simulink model "control_nonlinear"  (R2025a)
settings: Solver=VariableStepAuto  StartTime=0.0  StopTime=10.0  RelTol=1e-3
values from neighbouring files (symbols this model uses):
  dth1_0 = casos(k, 4)    [main.m]
  dth2_0 = casos(k, 6)    [main.m]
  dxc_0 = casos(k, 2)    [main.m]
  g = 9.8    [main.m]
  l1 = 0.42    [main.m]
  l2 = 0.191    [main.m]
  m1 = 3.0    (= 3)    [main.m]
  m2 = 3.3    [main.m]
  Mc = 5.5    [main.m]
  th1_0 = casos(k, 3)    [main.m]
  th2_0 = casos(k, 5)    [main.m]
  xc_0 = casos(k, 1)    [main.m]
undefined symbols (not defined in the file or in its folder): K, K_cancel, T, X, Y, Z
libraries: sm_lib x43, nesl_utility x10
(part 1 of 2)
settings Model: Creator=amoralesma  LastModifiedBy=amoralesma

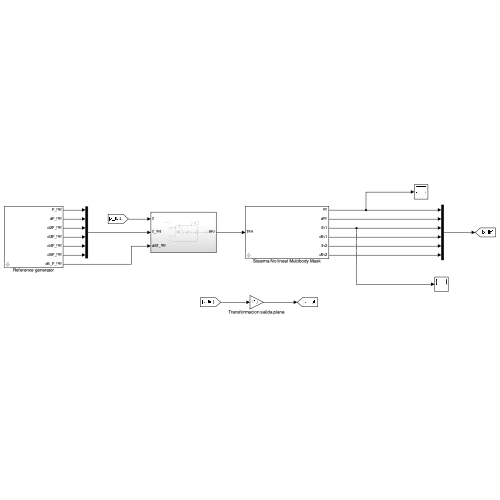
[thumbnail: Simulink's stored preview of the top-level diagram]
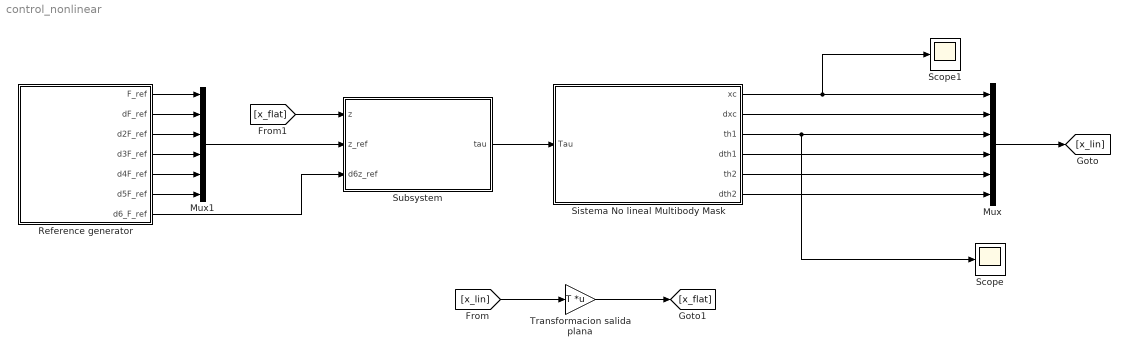
== system control_nonlinear ==
  Mux : Mux  Inputs=6
  Mux1 : Mux  Inputs=6
  Reference generator : Subsystem  mask(Generador señales de referencia carro y dos pendulos.){z2f=T, xc_in=xc_0, dxc_in=dxc_0, th1_in=th1_0, dth1_in=dth1_0, th2_in=th2_0, dth2_in=dth2_0, tf_=8, xc_f=-3, ref_config_sel=Suave quinta derivada (polinomio orden 11)}
      mask prompts: z2f "Matriz (6x6) transformación estados a salida plana"; tf_ "Tiempo final [s]"; xc_f "Posición final carro [m]"; ref_config_sel "Suavidad referencia"
      mask help: Este bloque realiza el planeamiento de las señales de referencia de las salida plana y sus derivadas, para un sistema de sexto orden, que corresponde a un carro con dos pendulos. Utiliza teoría de planitud diferencial y información de las condiciones iniciales y finales del sistema.
      mask init:
      | MaskNames = get_param(gcb,'MaskNames');
      | MaskVal = get_param(gcb,'MaskValues');
      | MaskObj = get_param(gcb,'MaskObject');
      | Model_folder=fileparts(which(gcs));
      | 
      | for ii_msk=1:length(MaskObj.Parameters)
      |     Obj_ii=MaskObj.Parameters(ii_msk);
      |     switch Obj_ii.Type
      |         case 'popup'
      |             eval([Obj_ii.Name,'=''',Obj_ii.Value,''';']);
      |             idx=find(strcmp(Obj_ii.TypeOptions, Obj_ii.Value));
      |             eval([Obj_ii.Name,'_idx=',num2str(idx),';']);
      |             clear idx  
      |         case 'edit'
      |             try
      |                 eval([MaskNames{ii_msk},'=',MaskVal{ii_msk},';']);
      |             catch
      |                 Work_space_vars=MaskObj.getWorkspaceVariables;
      |                idx_value=find(strcmp(MaskNames{ii_msk},{Work_space_vars.Name}));
      |                eval([MaskNames{ii_msk},'=Work_space_vars(idx_value).Value;'])
      |             end
      | 
      |         case 'checkbox'
      | 
      |             if strcmp(MaskVal{ii_msk},'on')
      |                 eval([MaskNames{ii_msk},'=true;']);
      |             else
      |                 eval([MaskNames{ii_msk},'=false;']);
      |             end
      | 
      |         case 'customtable'
      | 
      |             eval([MaskNames{ii_msk},'=',Obj_ii.Value,';']);
      |             eval([MaskNames{ii_msk},'_par=Obj_ii;']);
      |             eval([MaskNames{ii_msk},'_ctr=Obj_ii.DialogControl;']);
      | 
      |         case 'listbox'
      | 
      |             Options=Obj_ii.TypeOptions;
      |             if ~isempty(Obj_ii.TypeOptions)
      |                 if ~strcmp(Obj_ii.Value,'<empty>')
      |                     eval(['Val=',Obj_ii.Value,';'])
      |                     eval([MaskNames{ii_msk},'_idx=ismember(Options,Val);']);
      |                     eval([MaskNames{ii_msk},'=Options(ismember(Options,Val));']);
      |                 else
      |                     Val='<empty>';
      |                     eval([MaskNames{ii_msk},'_idx=ismember(Options,Val);']);
      |                     eval([MaskNames{ii_msk},'=Options(ismember(Options,Val));']);
      | 
      |                 end
      |             end
      | 
      |         case 'spinbox'
      | 
      |           
      |             eval([MaskNames{ii_msk},'=',MaskVal{ii_msk},';']);
      | 
      |     end      
      | end
      | 
      | 
      | t0_=0;
      | 
      | Coeff_nums=[2,4,6,8,10,12];
      | 
      | Coeff_num=Coeff_nums(ref_config_sel_idx);
      | 
      | 
      | z0_=[xc_in;dxc_in;th1_in;dth1_in;th2_in;dth2_in];
      | zf_=[xc_f;0;0;0;0;0];
      | 
      | F0_=z2f*z0_;
      | Ff_=z2f*zf_;
      | 
      | A_F=[1*t0_^11,      1*t0_^10,      1*t0_^9,        1*t0_^8,        1*t0_^7,        1*t0_^6,        1*t0_^5,   1*t0_^4,          1*t0_^3     1*t0_^2,    t0_,    1;...
      |      11*t0_^10,     10*t0_^9,      9*t0_^8,        8*t0_^7,        7*t0_^6,        6*t0_^5,        5*t0_^4,   4*t0_^3,          3*t0_^2     2*t0_^1,    1,      0;...
      |      110*t0_^9,     90*t0_^8,      72*t0_^7,       56*t0_^6,       42*t0_^5,       30*t0_^4,       20*t0_^3,  12*t0_^2,         6*t0_^1     2,          0,      0;...
      |      990*t0_^8,     720*t0_^7,     504*t0_^6,      336*t0_^5,      210*t0_^4,      120*t0_^3,      60*t0_^2,  24*t0_^1,         6           0,          0,      0;...
      |      7920*t0_^7,    5040*t0_^6,    3024*t0_^5,     1680*t0_^4,     840*t0_^3,      360*t0_^2,      120*t0_^1, 24,               0           0,          0,      0;...
      |      55440*t0_^6,   30240*t0_^5,   15120*t0_^4,    6720*t0_^3,     2520*t0_^2,     720*t0_^1,      120,       0,                0           0,          0,      0;...
      |      1*tf_^11,      1*tf_^10,      1*tf_^9,        1*tf_^8,        1*tf_^7,        1*tf_^6,        1*tf_^5,   1*tf_^4,          1*tf_^3     1*tf_^2,    tf_,    1;...
      |      11*tf_^10,     10*tf_^9,      9*tf_^8,        8*tf_^7,        7*tf_^6,        6*tf_^5,        5*tf_^4,   4*tf_^3,          3*tf_^2     2*tf_^1,    1,      0;...
      |      110*tf_^9,     90*tf_^8,      72*tf_^7,       56*tf_^6,       42*tf_^5,       30*tf_^4,       20*tf_^3,  12*tf_^2,         6*tf_^1     2,          0,      0;...
      |      990*tf_^8,     720*tf_^7,     504*tf_^6,      336*tf_^5,      210*tf_^4,      120*tf_^3,      60*tf_^2,  24*tf_^1,         6           0,          0,      0;...
      |      7920*tf_^7,    5040*tf_^6,    3024*tf_^5,     1680*tf_^4,     840*tf_^3,      360*tf_^2,      120*tf_^1, 24,               0           0,          0,      0;...
      |      55440*tf_^6,   30240*tf_^5,   15120*tf_^4,    6720*tf_^3,     2520*tf_^2,     720*tf_^1,      120,       0,                0           0,          0,      0];
      | 
      | A_F0=A_F(1:ref_config_sel_idx,end-Coeff_num+1:end);
      | A_Ff=A_F(7:6+ref_config_sel_idx,end-Coeff_num+1:end);
      | A_F_=[A_F0;A_Ff];
      | 
      | 
      | F_t0_tf=[F0_(1:ref_config_sel_idx);Ff_(1:ref_config_sel_idx)];
      | 
      | Pa=A_F_\F_t0_tf;
      | 
      | Pa_flip=flip(Pa);
      | size_Pa=size(Pa_flip,1);
      | for ii=0:11
      |     if ii+1<=size_Pa
      |         eval(['a',num2str(ii),'=Pa_flip(',num2str(ii+1),');'])
      |     else
      |         eval(['a',num2str(ii),'=0;'])
      |     end
      | end
      | 
      | 
      | PF_ref  =[a11,                  a10,                a9,             a8,             a7,             a6,             a5,             a4,         a3,         a2,     a1,     a0];
      | PdF_ref =[11*a11,               10*a10,             9*a9,           8*a8,           7*a7,           6*a6,           5*a5,           4*a4,       3*a3,       2*a2,   1*a1];
      | Pd2F_ref=[11*10*a11,            10*9*a10,           9*8*a9,         8*7*a8,         7*6*a7,         6*5*a6,         5*4*a5,         4*3*a4,     3*2*a3,     2*1*a2];
      | Pd3F_ref=[11*10*9*a11,          10*9*8*a10,         9*8*7*a9,       8*7*6*a8,       7*6*5*a7,       6*5*4*a6,       5*4*3*a5,       4*3*2*a4,   3*2*1*a3];
      | Pd4F_ref=[11*10*9*8*a11,        10*9*8*7*a10,       9*8*7*6*a9,     8*7*6*5*a8,     7*6*5*4*a7,     6*5*4*3*a6,     5*4*3*2*a5,     4*3*2*1*a4];
      | Pd5F_ref=[11*10*9*8*7*a11,      10*9*8*7*6*a10,     9*8*7*6*5*a9,   8*7*6*5*4*a8,   7*6*5*4*3*a7,   6*5*4*3*2*a6,   5*4*3*2*1*a5];
      | Pd6F_ref=[11*10*9*8*7*6*a11,    10*9*8*7*6*5*a10,   9*8*7*6*5*4*a9, 8*7*6*5*4*3*a8, 7*6*5*4*3*2*a7, 6*5*4*3*2*1*a6];
      | 
      | 
      | tsim_=linspace(t0_,tf_,10000);
      | 
      | 
      | d0F_ref   = polyval(PF_ref,tsim_);
      | d1F_ref  = polyval(PdF_ref,tsim_);
      | d2F_ref = polyval(Pd2F_ref,tsim_);
      | d3F_ref = polyval(Pd3F_ref,tsim_);
      | d4F_ref = polyval(Pd4F_ref,tsim_);
      | d5F_ref = polyval(Pd5F_ref,tsim_);
      | d6F_ref = polyval(Pd6F_ref,tsim_);
      | 
      | 
      | F_ref=[tsim_;d0F_ref;d1F_ref;d2F_ref;d3F_ref;d4F_ref;d5F_ref;d6F_ref]';
      mask TypeOptions ref_config_sel: Sin suavidad (polinomio orden 1) | Suave primera derivada (polinomio orden 3) | Suave segunda derivada (polinomio orden 5) | Suave tercera derivada (polinomio orden 7) | Suave cuarta derivada (polinomio orden 9) | Suave quinta derivada (polinomio orden 11)
      mask DialogControl Container_system Prompt: Información sistema
      mask DialogControl Container_init Prompt: Condiciones iniciales (t=0)
      mask DialogControl xc_in_lab Prompt: Posición inicial carro [m]
      mask DialogControl dxc_in_lab Prompt: Velocidad inicial carro [m/s]
      mask DialogControl th1_in_lab Prompt: Angulo inicial pendulo 1 [rad]
      mask DialogControl dth1_in_lab Prompt: Velocidad angular inicial pendulo 1 [rad/s]
      mask DialogControl th2_in_lab Prompt: Angulo inicial pendulo 2 [rad]
      mask DialogControl dth2_in_lab Prompt: Velocidad angular inicial pendulo 2 [rad/s]
      mask DialogControl Container_final Prompt: Condiciones finales (t=0)
      mask DialogControl Container_config Prompt: Configuración planeamiento
      mask DialogControl fig_f Prompt: Visualizar salida plana y derivadas
      mask DialogControl fig_f Callback:
      | MaskNames = get_param(gcb,'MaskNames');
      | MaskVal = get_param(gcb,'MaskValues');
      | MaskObj = get_param(gcb,'MaskObject');
      | Model_folder=fileparts(which(gcs));
      | 
      | for ii_msk=1:length(MaskObj.Parameters)
      |     Obj_ii=MaskObj.Parameters(ii_msk);
      |     switch Obj_ii.Type
      |         case 'popup'
      |             eval([Obj_ii.Name,'=''',Obj_ii.Value,''';']);
      |             idx=find(strcmp(Obj_ii.TypeOptions, Obj_ii.Value));
      |             eval([Obj_ii.Name,'_idx=',num2str(idx),';']);
      |             clear idx
      |         case 'edit'
      |             try
      |                 eval([MaskNames{ii_msk},'=',MaskVal{ii_msk},';']);
      |             catch
      |                 Work_space_vars=MaskObj.getWorkspaceVariables;
      |                idx_value=find(strcmp(MaskNames{ii_msk},{Work_space_vars.Name}));
      |                eval([MaskNames{ii_msk},'=Work_space_vars(idx_value).Value;'])
      |             end
      | 
      |         case 'checkbox'
      | 
      |             if strcmp(MaskVal{ii_msk},'on')
      |                 eval([MaskNames{ii_msk},'=true;']);
      |             else
      |                 eval([MaskNames{ii_msk},'=false;']);
      |             end
      | 
      |         case 'customtable'
      | 
      |             eval([MaskNames{ii_msk},'=',Obj_ii.Value,';']);
      |             eval([MaskNames{ii_msk},'_par=Obj_ii;']);
      |             eval([MaskNames{ii_msk},'_ctr=Obj_ii.DialogControl;']);
      | 
      |         case 'listbox'
      | 
      |             Options=Obj_ii.TypeOptions;
      |             if ~isempty(Obj_ii.TypeOptions)
      |                 if ~strcmp(Obj_ii.Value,'<empty>')
      |                     eval(['Val=',Obj_ii.Value,';'])
      |                     eval([MaskNames{ii_msk},'_idx=ismember(Options,Val);']);
      |                     eval([MaskNames{ii_msk},'=Options(ismember(Options,Val));']);
      |                 else
      |                     Val='<empty>';
      |                     eval([MaskNames{ii_msk},'_idx=ismember(Options,Val);']);
      |                     eval([MaskNames{ii_msk},'=Options(ismember(Options,Val));']);
      | 
      |                 end
      |             end
      | 
      |         case 'spinbox'
      | 
      | 
      |             eval([MaskNames{ii_msk},'=',MaskVal{ii_msk},';']);
      | 
      |     end
      | end
      | 
      | 
      | t0_=0;
      | 
      | Coeff_nums=[2,4,6,8,10,12];
      | 
      | Coeff_num=Coeff_nums(ref_config_sel_idx);
      | 
      | 
      | z0_=[xc_in;dxc_in;th1_in;dth1_in;th2_in;dth2_in];
      | zf_=[xc_f;0;0;0;0;0];
      | 
      | F0_=z2f*z0_;
      | Ff_=z2f*zf_;
      | 
      | A_F=[1*t0_^11,      1*t0_^10,      1*t0_^9,        1*t0_^8,        1*t0_^7,        1*t0_^6,        1*t0_^5,   1*t0_^4,          1*t0_^3     1*t0_^2,    t0_,    1;...
      |      11*t0_^10,     10*t0_^9,      9*t0_^8,        8*t0_^7,        7*t0_^6,        6*t0_^5,        5*t0_^4,   4*t0_^3,          3*t0_^2     2*t0_^1,    1,      0;...
      |      110*t0_^9,     90*t0_^8,      72*t0_^7,       56*t0_^6,       42*t0_^5,       30*t0_^4,       20*t0_^3,  12*t0_^2,         6*t0_^1     2,          0,      0;...
      |      990*t0_^8,     720*t0_^7,     504*t0_^6,      336*t0_^5,      210*t0_^4,      120*t0_^3,      60*t0_^2,  24*t0_^1,         6           0,          0,      0;...
      |      7920*t0_^7,    5040*t0_^6,    3024*t0_^5,     1680*t0_^4,     840*t0_^3,      360*t0_^2,      120*t0_^1, 24,               0           0,          0,      0;...
      |      55440*t0_^6,   30240*t0_^5,   15120*t0_^4,    6720*t0_^3,     2520*t0_^2,     720*t0_^1,      120,       0,                0           0,          0,      0;...
      |      1*tf_^11,      1*tf_^10,      1*tf_^9,        1*tf_^8,        1*tf_^7,        1*tf_^6,        1*tf_^5,   1*tf_^4,          1*tf_^3     1*tf_^2,    tf_,    1;...
      |      11*tf_^10,     10*tf_^9,      9*tf_^8,        8*tf_^7,        7*tf_^6,        6*tf_^5,        5*tf_^4,   4*tf_^3,          3*tf_^2     2*tf_^1,    1,      0;...
      |      110*tf_^9,     90*tf_^8,      72*tf_^7,       56*tf_^6,       42*tf_^5,       30*tf_^4,       20*tf_^3,  12*tf_^2,         6*tf_^1     2,          0,      0;...
      |      990*tf_^8,     720*tf_^7,     504*tf_^6,      336*tf_^5,      210*tf_^4,      120*tf_^3,      60*tf_^2,  24*tf_^1,         6           0,          0,      0;...
      |      7920*tf_^7,    5040*tf_^6,    3024*tf_^5,     1680*tf_^4,     840*tf_^3,      360*tf_^2,      120*tf_^1, 24,               0           0,          0,      0;...
      |      55440*tf_^6,   30240*tf_^5,   15120*tf_^4,    6720*tf_^3,     2520*tf_^2,     720*tf_^1,      120,       0,                0           0,          0,      0];
      | 
      | A_F0=A_F(1:ref_config_sel_idx,end-Coeff_num+1:end);
      | A_Ff=A_F(7:6+ref_config_sel_idx,end-Coeff_num+1:end);
      | A_F_=[A_F0;A_Ff];
      | 
      | 
      | F_t0_tf=[F0_(1:ref_config_sel_idx);Ff_(1:ref_config_sel_idx)];
      | 
      | Pa=A_F_\F_t0_tf;
      | 
      | Pa_flip=flip(Pa);
      | size_Pa=size(Pa_flip,1);
      | for ii=0:11
      |     if ii+1<=size_Pa
      |         eval(['a',num2str(ii),'=Pa_flip(',num2str(ii+1),');'])
      |     else
      |         eval(['a',num2str(ii),'=0;'])
      |     end
      | end
      | 
      | 
      | PF_ref  =[a11,                  a10,                a9,             a8,             a7,             a6,             a5,             a4,         a3,         a2,     a1,     a0];
      | PdF_ref =[11*a11,               10*a10,             9*a9,           8*a8,           7*a7,           6*a6,           5*a5,           4*a4,       3*a3,       2*a2,   1*a1];
      | Pd2F_ref=[11*10*a11,            10*9*a10,           9*8*a9,         8*7*a8,         7*6*a7,         6*5*a6,         5*4*a5,         4*3*a4,     3*2*a3,     2*1*a2];
      | Pd3F_ref=[11*10*9*a11,          10*9*8*a10,         9*8*7*a9,       8*7*6*a8,       7*6*5*a7,       6*5*4*a6,       5*4*3*a5,       4*3*2*a4,   3*2*1*a3];
      | Pd4F_ref=[11*10*9*8*a11,        10*9*8*7*a10,       9*8*7*6*a9,     8*7*6*5*a8,     7*6*5*4*a7,     6*5*4*3*a6,     5*4*3*2*a5,     4*3*2*1*a4];
      | Pd5F_ref=[11*10*9*8*7*a11,      10*9*8*7*6*a10,     9*8*7*6*5*a9,   8*7*6*5*4*a8,   7*6*5*4*3*a7,   6*5*4*3*2*a6,   5*4*3*2*1*a5];
      | Pd6F_ref=[11*10*9*8*7*6*a11,    10*9*8*7*6*5*a10,   9*8*7*6*5*4*a9, 8*7*6*5*4*3*a8, 7*6*5*4*3*2*a7, 6*5*4*3*2*1*a6];
      | 
      | 
      | tsim_=linspace(t0_,tf_,10000);
      | 
      | 
      | d0F_ref   = polyval(PF_ref,tsim_);
      | d1F_ref  = polyval(PdF_ref,tsim_);
      | d2F_ref = polyval(Pd2F_ref,tsim_);
      | d3F_ref = polyval(Pd3F_ref,tsim_);
      | d4F_ref = polyval(Pd4F_ref,tsim_);
      | d5F_ref = polyval(Pd5F_ref,tsim_);
      | d6F_ref = polyval(Pd6F_ref,tsim_);
      | 
      | figure('Color',[1,1,1])
      | set(groot,'defaultAxesTickLabelInterpreter','latex');
      | set(groot,'defaulttextinterpreter','latex');
      | set(groot,'defaultLegendInterpreter','latex');
      | 
      | ax_01=subplot(7,1,1);
      | hold on
      | grid on
      | 
      | ylabel('$f_{ref}(t)$','FontName','Times New Roman','FontAngle','normal','FontWeight','bold','FontSize',15)
      | 
      | ax_02=subplot(7,1,2);
      | 
      | ylabel('$f_{ref}''(t)$','FontName','Times New Roman','FontAngle','normal','FontWeight','bold','FontSize',15)
      | hold on
      | grid on
      | 
      | ax_03=subplot(7,1,3);
      | 
      | ylabel('$f_{ref}''''(t)$','FontName','Times New Roman','FontAngle','normal','FontWeight','bold','FontSize',15)
      | hold on
      | grid on
      | 
      | ax_04=subplot(7,1,4);
      | 
      | ylabel('$f_{ref}''''''(t)$','FontName','Times New Roman','FontAngle','normal','FontWeight','bold','FontSize',15)
      | hold on
      | grid on
      | ax_05=subplot(7,1,5);
      | 
      | ylabel('$f_{ref}^{(4)}(t)$','FontName','Times New Roman','FontAngle','normal','FontWeight','bold','FontSize',15)
      | hold on
      | grid on
      | 
      | ax_06=subplot(7,1,6);
      | 
      | ylabel('$f_{ref}^{(5)}(t)$','FontName','Times New Roman','FontAngle','normal','FontWeight','bold','FontSize',15)
      | hold on
      | grid on
      | 
      | ax_07=subplot(7,1,7);
      | 
      | ylabel('$f_{ref}^{(6)}(t)$','FontName','Times New Roman','FontAngle','normal','FontWeight','bold','FontSize',15)
      | xlabel('Tiempo [s]','FontName','Times New Roman','FontAngle','normal','FontWeight','bold','FontSize',15)
      | hold on
      | grid on
      | 
      | plot(ax_01,tsim_,d0F_ref,'Color','k')
      | plot(ax_01,0,F0_(1),'Color','r','Marker','o')
      | plot(ax_01,tf_,Ff_(1),'Color','b','Marker','x')
      | 
      | plot(ax_02,tsim_,d1F_ref,'Color','k')
      | plot(ax_02,0,F0_(2),'Color','r','Marker','o')
      | plot(ax_02,tf_,Ff_(2),'Color','b','Marker','x')
      | 
      | plot(ax_03,tsim_,d2F_ref,'Color','k')
      | plot(ax_03,0,F0_(3),'Color','r','Marker','o')
      | plot(ax_03,tf_,Ff_(3),'Color','b','Marker','x')
      | 
      | plot(ax_04,tsim_,d3F_ref,'Color','k')
      | plot(ax_04,0,F0_(4),'Color','r','Marker','o')
      | plot(ax_04,tf_,Ff_(4),'Color','b','Marker','x')
      | 
      | plot(ax_05,tsim_,d4F_ref,'Color','k')
      | plot(ax_05,0,F0_(5),'Color','r','Marker','o')
      | plot(ax_05,tf_,Ff_(5),'Color','b','Marker','x')
      | 
      | plot(ax_06,tsim_,d5F_ref,'Color','k')
      | plot(ax_06,0,F0_(6),'Color','r','Marker','o')
      | plot(ax_06,tf_,Ff_(6),'Color','b','Marker','x')
      | 
      | plot(ax_07,tsim_,d6F_ref,'Color','k')
      | 
      | sgtitle('Referencia salida plana y derivadas');
      mask DialogControl fig_z Prompt: Visualizar estados
      mask DialogControl fig_z Callback:
      | MaskNames = get_param(gcb,'MaskNames');
      | MaskVal = get_param(gcb,'MaskValues');
      | MaskObj = get_param(gcb,'MaskObject');
      | Model_folder=fileparts(which(gcs));
      | 
      | for ii_msk=1:length(MaskObj.Parameters)
      |     Obj_ii=MaskObj.Parameters(ii_msk);
      |     switch Obj_ii.Type
      |         case 'popup'
      |             eval([Obj_ii.Name,'=''',Obj_ii.Value,''';']);
      |             idx=find(strcmp(Obj_ii.TypeOptions, Obj_ii.Value));
      |             eval([Obj_ii.Name,'_idx=',num2str(idx),';']);
      |             clear idx
      |         case 'edit'
      |             try
      |                 eval([MaskNames{ii_msk},'=',MaskVal{ii_msk},';']);
      |             catch
      |                 Work_space_vars=MaskObj.getWorkspaceVariables;
      |                idx_value=find(strcmp(MaskNames{ii_msk},{Work_space_vars.Name}));
      |                eval([MaskNames{ii_msk},'=Work_space_vars(idx_value).Value;'])
      |             end
      | 
      |         case 'checkbox'
      | 
      |             if strcmp(MaskVal{ii_msk},'on')
      |                 eval([MaskNames{ii_msk},'=true;']);
      |             else
      |                 eval([MaskNames{ii_msk},'=false;']);
      |             end
      | 
      |         case 'customtable'
      | 
      |             eval([MaskNames{ii_msk},'=',Obj_ii.Value,';']);
      |             eval([MaskNames{ii_msk},'_par=Obj_ii;']);
      |             eval([MaskNames{ii_msk},'_ctr=Obj_ii.DialogControl;']);
      | 
      |         case 'listbox'
      | 
      |             Options=Obj_ii.TypeOptions;
      |             if ~isempty(Obj_ii.TypeOptions)
      |                 if ~strcmp(Obj_ii.Value,'<empty>')
      |                     eval(['Val=',Obj_ii.Value,';'])
      |                     eval([MaskNames{ii_msk},'_idx=ismember(Options,Val);']);
      |                     eval([MaskNames{ii_msk},'=Options(ismember(Options,Val));']);
      |                 else
      |                     Val='<empty>';
      |                     eval([MaskNames{ii_msk},'_idx=ismember(Options,Val);']);
      |                     eval([MaskNames{ii_msk},'=Options(ismember(Options,Val));']);
      | 
      |                 end
      |             end
      | 
      |         case 'spinbox'
      | 
      | 
      |             eval([MaskNames{ii_msk},'=',MaskVal{ii_msk},';']);
      | 
      |     end
      | end
      | 
      | 
      | t0_=0;
      | 
      | Coeff_nums=[2,4,6,8,10,12];
      | 
      | Coeff_num=Coeff_nums(ref_config_sel_idx);
      | 
      | 
      | z0_=[xc_in;dxc_in;th1_in;dth1_in;th2_in;dth2_in];
      | zf_=[xc_f;0;0;0;0;0];
      | 
      | F0_=z2f*z0_;
      | Ff_=z2f*zf_;
      | 
      | A_F=[1*t0_^11,      1*t0_^10,      1*t0_^9,        1*t0_^8,        1*t0_^7,        1*t0_^6,        1*t0_^5,   1*t0_^4,          1*t0_^3     1*t0_^2,    t0_,    1;...
      |      11*t0_^10,     10*t0_^9,      9*t0_^8,        8*t0_^7,        7*t0_^6,        6*t0_^5,        5*t0_^4,   4*t0_^3,          3*t0_^2     2*t0_^1,    1,      0;...
      |      110*t0_^9,     90*t0_^8,      72*t0_^7,       56*t0_^6,       42*t0_^5,       30*t0_^4,       20*t0_^3,  12*t0_^2,         6*t0_^1     2,          0,      0;...
      |      990*t0_^8,     720*t0_^7,     504*t0_^6,      336*t0_^5,      210*t0_^4,      120*t0_^3,      60*t0_^2,  24*t0_^1,         6           0,          0,      0;...
      |      7920*t0_^7,    5040*t0_^6,    3024*t0_^5,     1680*t0_^4,     840*t0_^3,      360*t0_^2,      120*t0_^1, 24,               0           0,          0,      0;...
      |      55440*t0_^6,   30240*t0_^5,   15120*t0_^4,    6720*t0_^3,     2520*t0_^2,     720*t0_^1,      120,       0,                0           0,          0,      0;...
      |      1*tf_^11,      1*tf_^10,      1*tf_^9,        1*tf_^8,        1*tf_^7,        1*tf_^6,        1*tf_^5,   1*tf_^4,          1*tf_^3     1*tf_^2,    tf_,    1;...
      |      11*tf_^10,     10*tf_^9,      9*tf_^8,        8*tf_^7,        7*tf_^6,        6*tf_^5,        5*tf_^4,   4*tf_^3,          3*tf_^2     2*tf_^1,    1,      0;...
      |      110*tf_^9,     90*tf_^8,      72*tf_^7,       56*tf_^6,       42*tf_^5,       30*tf_^4,       20*tf_^3,  12*tf_^2,         6*tf_^1     2,          0,      0;...
      |      990*tf_^8,     720*tf_^7,     504*tf_^6,      336*tf_^5,      210*tf_^4,      120*tf_^3,      60*tf_^2,  24*tf_^1,         6           0,          0,      0;...
      |      7920*tf_^7,    5040*tf_^6,    3024*tf_^5,     1680*tf_^4,     840*tf_^3,      360*tf_^2,      120*tf_^1, 24,               0           0,          0,      0;...
      |      55440*tf_^6,   30240*tf_^5,   15120*tf_^4,    6720*tf_^3,     2520*tf_^2,     720*tf_^1,      120,       0,                0           0,          0,      0];
      | 
      | A_F0=A_F(1:ref_config_sel_idx,end-Coeff_num+1:end);
      | A_Ff=A_F(7:6+ref_config_sel_idx,end-Coeff_num+1:end);
      | A_F_=[A_F0;A_Ff];
      | 
      | 
      | F_t0_tf=[F0_(1:ref_config_sel_idx);Ff_(1:ref_config_sel_idx)];
      | 
      | Pa=A_F_\F_t0_tf;
      | 
      | Pa_flip=flip(Pa);
      | size_Pa=size(Pa_flip,1);
      | for ii=0:11
      |     if ii+1<=size_Pa
      |         eval(['a',num2str(ii),'=Pa_flip(',num2str(ii+1),');'])
      |     else
      |         eval(['a',num2str(ii),'=0;'])
      |     end
      | end
      | 
      | 
      | PF_ref  =[a11,                  a10,                a9,             a8,             a7,             a6,             a5,             a4,         a3,         a2,     a1,     a0];
      | PdF_ref =[11*a11,               10*a10,             9*a9,           8*a8,           7*a7,           6*a6,           5*a5,           4*a4,       3*a3,       2*a2,   1*a1];
      | Pd2F_ref=[11*10*a11,            10*9*a10,           9*8*a9,         8*7*a8,         7*6*a7,         6*5*a6,         5*4*a5,         4*3*a4,     3*2*a3,     2*1*a2];
      | Pd3F_ref=[11*10*9*a11,          10*9*8*a10,         9*8*7*a9,       8*7*6*a8,       7*6*5*a7,       6*5*4*a6,       5*4*3*a5,       4*3*2*a4,   3*2*1*a3];
      | Pd4F_ref=[11*10*9*8*a11,        10*9*8*7*a10,       9*8*7*6*a9,     8*7*6*5*a8,     7*6*5*4*a7,     6*5*4*3*a6,     5*4*3*2*a5,     4*3*2*1*a4];
      | Pd5F_ref=[11*10*9*8*7*a11,      10*9*8*7*6*a10,     9*8*7*6*5*a9,   8*7*6*5*4*a8,   7*6*5*4*3*a7,   6*5*4*3*2*a6,   5*4*3*2*1*a5];
      | Pd6F_ref=[11*10*9*8*7*6*a11,    10*9*8*7*6*5*a10,   9*8*7*6*5*4*a9, 8*7*6*5*4*3*a8, 7*6*5*4*3*2*a7, 6*5*4*3*2*1*a6];
      | 
      | 
      | tsim_=linspace(t0_,tf_,10000);
      | 
      | 
      | d0F_ref   = polyval(PF_ref,tsim_);
      | d1F_ref  = polyval(PdF_ref,tsim_);
      | d2F_ref = polyval(Pd2F_ref,tsim_);
      | d3F_ref = polyval(Pd3F_ref,tsim_);
      | d4F_ref = polyval(Pd4F_ref,tsim_);
      | d5F_ref = polyval(Pd5F_ref,tsim_);
      | d6F_ref = polyval(Pd6F_ref,tsim_);
      | 
      | 
      | F_total=[d0F_ref;d1F_ref;d2F_ref;d3F_ref;d4F_ref;d5F_ref];
      | f2z=inv(z2f);
      | z_total=f2z*F_total;
      | 
      | set(groot,'defaultAxesTickLabelInterpreter','latex');
      | set(groot,'defaulttextinterpreter','latex');
      | set(groot,'defaultLegendInterpreter','latex');
      | 
      | figure('Color',[1,1,1])
      | 
      | sgtitle('Referencia estados carro');
      | 
      | 
      | ax_01=subplot(2,1,1);
      | 
      | ylabel('$xc_{ref}(t) [m]$','FontName','Times New Roman','FontAngle','normal','FontWeight','bold','FontSize',15)
      | xlabel('Tiempo [s]','FontName','Times New Roman','FontAngle','normal','FontWeight','bold','FontSize',15)
      | hold on
      | grid on
      | 
      | 
      | ax_02=subplot(2,1,2);
      | 
      | ylabel('$\dot{x}c_{ref}(t) [m/s]$','FontName','Times New Roman','FontAngle','normal','FontWeight','bold','FontSize',15)
      | xlabel('Tiempo [s]','FontName','Times New Roman','FontAngle','normal','FontWeight','bold','FontSize',15)
      | hold on
      | grid on
      | 
      | figure('Color',[1,1,1])
      | sgtitle('Referencia estados pendulo 1');
      | 
      | ax_03=subplot(2,1,1);
      | 
      | xlabel('Tiempo [s]','FontName','Times New Roman','FontAngle','normal','FontWeight','bold','FontSize',15)
      | ylabel('$\theta_{1-ref}(t)[^{\circ}]$','FontName','Times New Roman','FontAngle','normal','FontWeight','bold','FontSize',15)
      | hold on
      | grid on
      | 
      | ax_04=subplot(2,1,2);
      | 
      | xlabel('Tiempo [s]','FontName','Times New Roman','FontAngle','normal','FontWeight','bold','FontSize',15)
      | ylabel('$\dot{\theta}_{1-ref}(t)[^{\circ}/s]$','FontName','Times New Roman','FontAngle','normal','FontWeight','bold','FontSize',15)
      | hold on
      | grid on
      | 
      | figure('Color',[1,1,1])
      | sgtitle('Referencia estados pendulo 2');
      | 
      | 
      | ax_05=subplot(2,1,1);
      | 
      | xlabel('Tiempo [s]','FontName','Times New Roman','FontAngle','normal','FontWeight','bold','FontSize',15)
      | ylabel('$\theta_{2-ref}(t)[^{\circ}]$','FontName','Times New Roman','FontAngle','normal','FontWeight','bold','FontSize',15)
      | hold on
      | grid on
      | 
      | ax_06=subplot(2,1,2);
      | 
      | xlabel('Tiempo [s]','FontName','Times New Roman','FontAngle','normal','FontWeight','bold','FontSize',15)
      | ylabel('$\dot{\theta}_{2-ref}(t)[^{\circ}/s]$','FontName','Times New Roman','FontAngle','normal','FontWeight','bold','FontSize',15)
      | 
      | hold on
      | grid on
      | 
      | plot(ax_01,tsim_,z_total(1,:),'Color','k')
      | plot(ax_01,0,z0_(1),'Color','r','Marker','o')
      | plot(ax_01,tf_,zf_(1),'Color','b','Marker','x')
      | 
      | plot(ax_02,tsim_,z_total(2,:),'Color','k')
      | plot(ax_02,0,z0_(2),'Color','r','Marker','o')
      | plot(ax_02,tf_,zf_(2),'Color','b','Marker','x')
      | 
      | plot(ax_03,tsim_,z_total(3,:)*180/pi,'Color','k')
      | plot(ax_03,0,z0_(3)*180/pi,'Color','r','Marker','o')
      | plot(ax_03,tf_,zf_(3)*180/pi,'Color','b','Marker','x')
      | 
      | plot(ax_04,tsim_,z_total(4,:)*180/pi,'Color','k')
      | plot(ax_04,0,z0_(4)*180/pi,'Color','r','Marker','o')
      | plot(ax_04,tf_,zf_(4)*180/pi,'Color','b','Marker','x')
      | 
      | plot(ax_05,tsim_,z_total(5,:)*180/pi,'Color','k')
      | plot(ax_05,0,z0_(5)*180/pi,'Color','r','Marker','o')
      | plot(ax_05,tf_,zf_(5)*180/pi,'Color','b','Marker','x')
      | 
      | plot(ax_06,tsim_,z_total(6,:)*180/pi,'Color','k')
      | plot(ax_06,0,z0_(6)*180/pi,'Color','r','Marker','o')
      | plot(ax_06,tf_,zf_(6)*180/pi,'Color','b','Marker','x')
  Scope : Scope
      settings: ActiveDisplayYMinimum=-20.355365048189331  ActiveDisplayYMaximum=62.467486682636242  DataLoggingVariableName=ScopeData2
  Scope1 : Scope
      settings: ActiveDisplayYMinimum=-991.47778994476  ActiveDisplayYMaximum=110.56541104410231  DataLoggingVariableName=ScopeData3
  Sistema No lineal Multibody Mask : Subsystem  mask(Carro pendulo doble){Mc=Mc, m1=m1, m2=m2, L1=l1, L2=l2, g=g, m_bar1=1e-9, m_bar2=1e-9, bc=0, b1=0, b2=0, xc_in=xc_0, dxc_in=dxc_0, th1_in=th1_0, dth1_in=dth1_0, th2_in=th2_0, dth2_in=dth2_0, bool_f_ext=off}
      mask prompts: Mc "Masa Carro [kg]"; m1 "Masa pendulo 1 [kg]"; m2 "Masa pendulo 2 [kg]"; L1 "Longitud barra 1 [m]"; L2 "Longitud barra 2 [m]"; g "Gravedad [m/s^2]"; m_bar1 "Masa barra 1 [kg]"; m_bar2 "Masa barra 2 [kg]"; bc "Amortiguamiento Carro [N/(m/s)]"; b1 "Amortiguamiento pendulo 1 [N*m/(rad/s)]"; b2 "Amortiguamiento pendulo 2 [N*m/(rad/s)]"; xc_in "Posición carro [m]"; dxc_in "Velocidad carro [m/s]"; th1_in "Angulo pendulo 1 [rad]"; dth1_in "Velocidad angular pendulo 1 [rad/s]"; th2_in "Angulo pendulo 2 [rad]"; dth2_in "Velocidad angular pendulo 2 [rad/s]"; bool_f_ext "Puerto fuerza horizontal en masa 1 o 2 [N]"
      mask help: Bloque de carro con doble pendulo diseñado para la asignatura de temas especiales de control Unal.
      mask init:
      | MaskNames = get_param(gcb,'MaskNames');
      | MaskVal = get_param(gcb,'MaskValues');
      | MaskObj = get_param(gcb,'MaskObject');
      | Model_folder=fileparts(which(gcs));
      | 
      | for ii_msk=1:length(MaskObj.Parameters)
      |     Obj_ii=MaskObj.Parameters(ii_msk);
      |     switch Obj_ii.Type
      |         case 'popup'
      |             eval([Obj_ii.Name,'=''',Obj_ii.Value,''';']);
      |             idx=find(strcmp(Obj_ii.TypeOptions, Obj_ii.Value));
      |             eval([Obj_ii.Name,'_idx=',num2str(idx),';']);
      |             clear idx  
      |         case 'edit'
      |             try
      |                 eval([MaskNames{ii_msk},'=',MaskVal{ii_msk},';']);
      |             catch
      |                 Work_space_vars=MaskObj.getWorkspaceVariables;
      |                idx_value=find(strcmp(MaskNames{ii_msk},{Work_space_vars.Name}));
      |                eval([MaskNames{ii_msk},'=Work_space_vars(idx_value).Value;'])
      |             end
      | 
      |         case 'checkbox'
      | 
      |             if strcmp(MaskVal{ii_msk},'on')
      |                 eval([MaskNames{ii_msk},'=true;']);
      |             else
      |                 eval([MaskNames{ii_msk},'=false;']);
      |             end
      | 
      |         case 'customtable'
      | 
      |             eval([MaskNames{ii_msk},'=',Obj_ii.Value,';']);
      |             eval([MaskNames{ii_msk},'_par=Obj_ii;']);
      |             eval([MaskNames{ii_msk},'_ctr=Obj_ii.DialogControl;']);
      | 
      |         case 'listbox'
      | 
      |             Options=Obj_ii.TypeOptions;
      |             if ~isempty(Obj_ii.TypeOptions)
      |                 if ~strcmp(Obj_ii.Value,'<empty>')
      |                     eval(['Val=',Obj_ii.Value,';'])
      |                     eval([MaskNames{ii_msk},'_idx=ismember(Options,Val);']);
      |                     eval([MaskNames{ii_msk},'=Options(ismember(Options,Val));']);
      |                 else
      |                     Val='<empty>';
      |                     eval([MaskNames{ii_msk},'_idx=ismember(Options,Val);']);
      |                     eval([MaskNames{ii_msk},'=Options(ismember(Options,Val));']);
      | 
      |                 end
      |             end
      | 
      |         case 'spinbox'
      | 
      |           
      |             eval([MaskNames{ii_msk},'=',MaskVal{ii_msk},';']);
      | 
      |     end      
      | end
      | 
      | input_blocks=[{[gcb,'/Input F1']},{[gcb,'/Input F2']}];
      | 
      | for ii=1:length(input_blocks)
      |     block_ii=input_blocks{ii};
      |     try
      |         block_type=get_param(block_ii, 'BlockType');
      |         if strcmp(block_type,'Inport') 
      |             if ~bool_f_ext
      |                 pos_ii=get_param(block_ii,'Position');
      |                 delete_block(block_ii)
      |                 add_block('simulink/Sources/Ground',block_ii)
      |                 set_param(block_ii,'Position',pos_ii)
      |             end
      |         else strcmp(block_type,'Ground') 
      |             if bool_f_ext
      |                 pos_ii=get_param(block_ii,'Position');
      |                 delete_block(block_ii)
      |                 add_block('simulink/Sources/In1',block_ii)
      |                 set_param(block_ii,'Position',pos_ii)
      |             end
      |         end
      |     end
      | end
      mask DialogControl Container_params Prompt: Parametros sistema
      mask DialogControl Container_params_sim Prompt: Parametros basicos
      mask DialogControl Container_params_adicionales Prompt: Parametros adicionales
      mask DialogControl Container_init Prompt: Condiciones iniciales
      mask DialogControl Container_inputs Prompt: Perturbaciones del sistema
  Subsystem : Subsystem
  Transformacion salida plana : Gain  Gain=T  Multiplication=Matrix(K*u)
  wires:
  Mux/1 -> [x_lin]
  [x_lin] -> Transformacion salida plana/1
  Transformacion salida plana/1 -> [x_flat]
  Subsystem/1(tau) -> Sistema No lineal Multibody Mask/1(Tau)
  Reference generator/1(F_ref) -> Mux1/1
  Reference generator/2(dF_ref) -> Mux1/2
  Reference generator/3(d2F_ref) -> Mux1/3
  Reference generator/4(d3F_ref) -> Mux1/4
  Reference generator/5(d4F_ref) -> Mux1/5
  Reference generator/6(d5F_ref) -> Mux1/6
  Mux1/1 -> Subsystem/2(z_ref)
  Reference generator/7(d6_F_ref) -> Subsystem/3(d6z_ref)
  [x_flat] -> Subsystem/1(z)
  Sistema No lineal Multibody Mask/1(xc) -> Scope1/1, Mux/1
  Sistema No lineal Multibody Mask/2(dxc) -> Mux/2
  Sistema No lineal Multibody Mask/3(th1) -> Scope/1, Mux/3
  Sistema No lineal Multibody Mask/4(dth1) -> Mux/4
  Sistema No lineal Multibody Mask/5(th2) -> Mux/5
  Sistema No lineal Multibody Mask/6(dth2) -> Mux/6

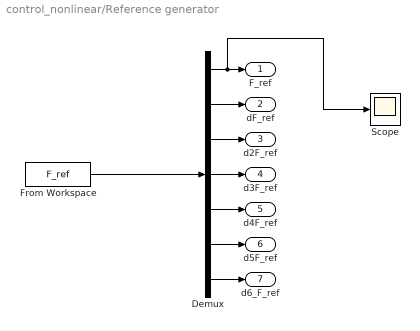
== system control_nonlinear/Reference generator ==
  Demux : Demux  Outputs=7
  From Workspace : FromWorkspace  VariableName=F_ref  OutputAfterFinalValue=Holding final value
  Scope : Scope
      settings: ActiveDisplayYMinimum=-1  ActiveDisplayYMaximum=1
  F_ref : Outport
  dF_ref : Outport  Port=2
  d2F_ref : Outport  Port=3
  d3F_ref : Outport  Port=4
  d4F_ref : Outport  Port=5
  d5F_ref : Outport  Port=6
  d6_F_ref : Outport  Port=7
  wires:
  From Workspace/1 -> Demux/1
  Demux/1 -> Scope/1, F_ref/1
  Demux/2 -> dF_ref/1
  Demux/3 -> d2F_ref/1
  Demux/4 -> d3F_ref/1
  Demux/5 -> d4F_ref/1
  Demux/6 -> d5F_ref/1
  Demux/7 -> d6_F_ref/1
